simulink model "model_motor"  (R2021b)
settings: Solver=ode45  StartTime=0.0  StopTime=20.0  RelTol=1e-3  EnableMultiTasking=on
undefined symbols (not defined in the file or in its folder): B, J, Ka, Km, L, Q, R
settings Model: Creator=The MathWorks, Inc.  LastModifiedBy=ulbio
settings SolverCC: AlgebraicLoopSolver=TrustRegion
settings DataIOCC: SaveFormat=Array  ReturnWorkspaceOutputs=off
settings OptimizationCC: BlockReduction=off  BooleanDataType=off  InitFltsAndDblsToZero=on  LifeSpan=inf
settings DebuggingCC: SaveWithParameterizedLinksMsg=none  UnderspecifiedInitializationDetection=Classic  MergeDetectMultiDrivingBlocksExec=none  SignalResolutionControl=TryResolveAllWithWarning  MultiTaskDSMMsg=warning  MultiTaskCondExecSysMsg=none  FcnCallInpInsideContextMsg=warning  SFUnexpectedBacktrackingDiag=warning  SFNoUnconditionalDefaultTransitionDiag=warning  SFExecutionAtInitializationDiag=none  SFMachineParentedDataDiag=warning  ArithmeticOperatorsInVariantConditions=warning
settings HardwareCC: ProdBitPerPointer=32  ProdBitPerSizeT=32  ProdBitPerPtrDiffT=32  ProdLargestAtomicFloat=None  ProdIntDivRoundTo=Undefined  ProdEndianess=Unspecified  ProdWordSize=32  ProdHWDeviceType=32-bit Generic  TargetUnknown=on
settings ModelReferenceCC: PropagateSignalLabelsOutOfModel=off
settings CodeAppCC: StateflowObjectComments=on
settings GRTTargetCC: TargetFcnLib=ansi_tfl_tmw.mat  TargetLangStandard=C89/C90 (ANSI)  CombineOutputUpdateFcns=off  GRTInterface=on
settings ConfigComp: CovMetricSettings=dw  CovSaveCumulativeToWorkspaceVar=on  CovSaveSingleToWorkspaceVar=on

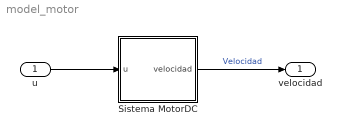
== system model_motor ==
  u : Inport
  Sistema MotorDC : Subsystem
  velocidad : Outport
  wires:
  u/1 -> Sistema MotorDC/1(u)
  Sistema MotorDC/1(velocidad) -> velocidad/1  "Velocidad"

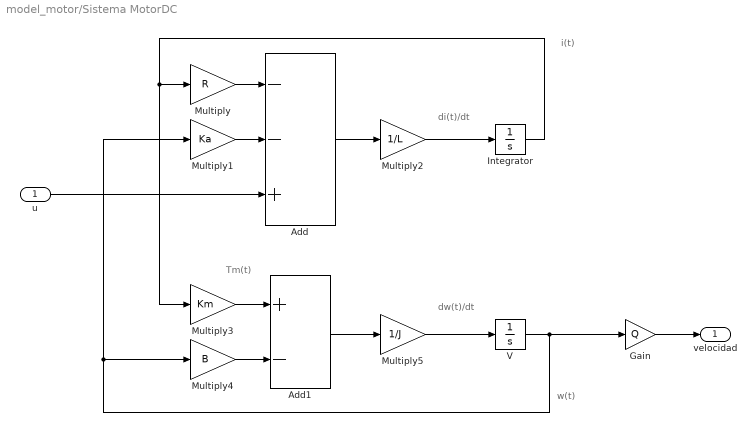
== system model_motor/Sistema MotorDC ==
  note: di(t)/dt
  note: w(t)
  note: Tm(t)
  note: i(t)
  note: dw(t)/dt
  u : Inport
  Add : Sum  Inputs=--+
  Add1 : Sum  Inputs=+-
  Gain : Gain  Gain=Q
  Integrator : Integrator
  Multiply : Gain  Gain=R
  Multiply1 : Gain  Gain=Ka
  Multiply2 : Gain  Gain=1/L
  Multiply3 : Gain  Gain=Km
  Multiply4 : Gain  Gain=B
  Multiply5 : Gain  Gain=1/J
  V : Integrator  LimitOutput=on  LowerSaturationLimit=0
  velocidad : Outport  VectorParamsAs1DForOutWhenUnconnected=off
  wires:
  Gain/1 -> velocidad/1
  Integrator/1 -> Multiply3/1, Multiply/1
  Multiply3/1 -> Add1/1
  u/1 -> Add/3
  Multiply2/1 -> Integrator/1
  Multiply1/1 -> Add/2
  Multiply4/1 -> Add1/2
  Add/1 -> Multiply2/1
  Multiply5/1 -> V/1
  V/1 -> Gain/1, Multiply1/1, Multiply4/1
  Multiply/1 -> Add/1
  Add1/1 -> Multiply5/1
